simulink model "velocity_feedback"  (R2023b)
settings: Solver=VariableStepAuto  StartTime=0.0  StopTime=10.0  RelTol=1e-3
libraries: cstblocks x4
settings Model: Creator=frenci  LastModifiedBy=frenci

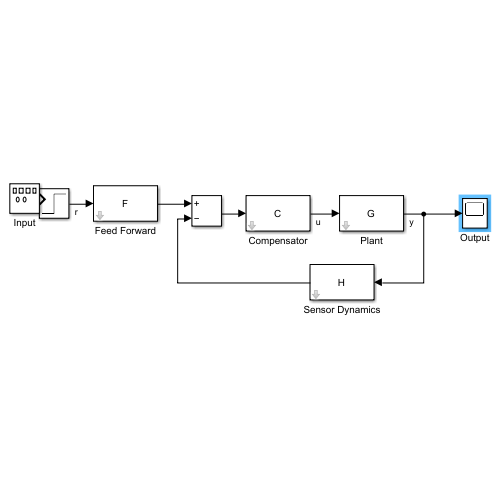
[thumbnail: Simulink's stored preview of the top-level diagram]
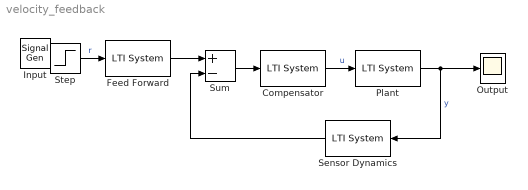
== system velocity_feedback ==
  Compensator : cstblocks/LTI System  sys=C  IC=[]  PadeOrder=0
  Feed Forward : cstblocks/LTI System  sys=F  IC=[]  PadeOrder=0
  Input : SignalGenerator
  Output : Scope
  Plant : cstblocks/LTI System  sys=G  IC=[]  PadeOrder=0
  Sensor Dynamics : cstblocks/LTI System  sys=H  IC=[]  PadeOrder=0
  Step : Step  SampleTime=0
  Sum : Sum  Inputs=+-
  wires:
  Step/1 -> Feed Forward/1  "r"
  Feed Forward/1 -> Sum/1
  Sensor Dynamics/1 -> Sum/2
  Sum/1 -> Compensator/1
  Compensator/1 -> Plant/1  "u"
  Plant/1 -> Output/1, Sensor Dynamics/1  "y"
